simulink library "ecrobot_nxt_lib"  (Simulink 6.4)
undefined symbols (not defined in the file or in its folder): BatteryVoltage, clearNXTSignalObjects, CompassSensorS1, EnterButton, GyroSensorS1, InitAccessorBlock, InitInterfaceBlock, LightSensorS1, RevolutionSensorA, RunButton, ServoMotorA, set_fcncallname, sfunxymap2, SoundSensorS1, SoundWAV, SystemClock, TouchSensorS1, TRACK_MAP, UltrasonicSensorS1
(part 1 of 2)
settings Model: Creator=tchikama  LastModifiedBy=tchikama

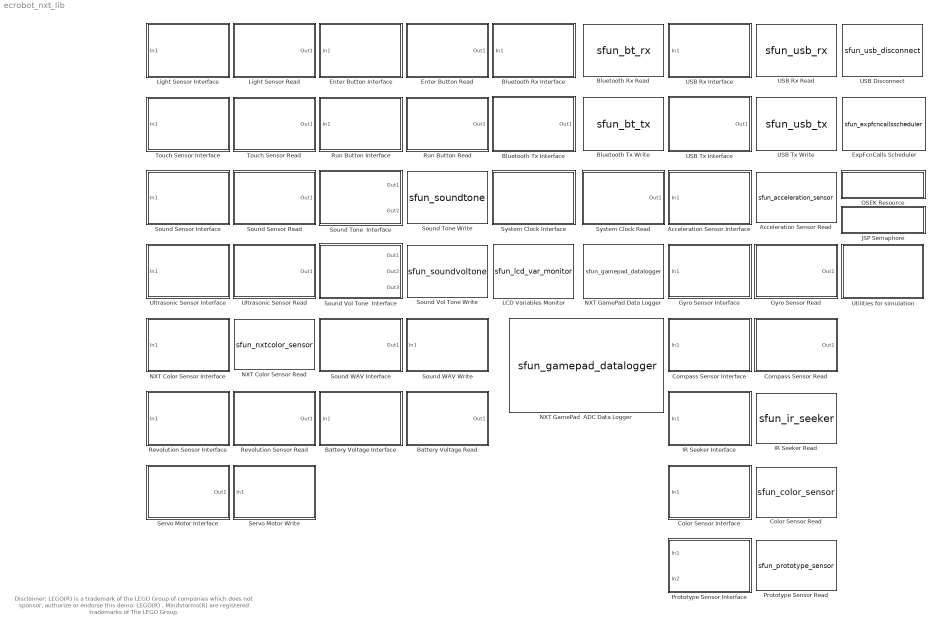
== system ecrobot_nxt_lib ==
  note: Disclaimer:
      | LEGO(R) is a trademark of the LEGO Group of companies which does not sponsor, authorize or endorse this demo.
      | LEGO(R) , Mindstorms(R) are registered trademarks of The LEGO Group.
  Acceleration Sensor Interface : Subsystem  StopFcn=clearNXTSignalObjects();  TreatAsAtomicUnit=on  mask(Acceleration Sensor Interface){ip=S1}
      mask prompts: ip "Port:"
      mask help:
      | HiTechnic Acceleration Sensor Interface for LEGO Mindstorms NXT.
      | Input is a vectorized signal:
      |  Index1: X axis acceleration
      |  Index2: Y axis acceleration
      |  Index3: Z axis acceleration
      | This block should be allocated outside of a Subsystem for RTW code generation.
      mask StyleString: popup(S1|S2|S3|S4)
      mask Display:
      | image(imread('HiTechnicSensor.jpg'))
      | port_label('input', 1, ['S' num2str(ip)])
  Acceleration Sensor Read : S-Function  FunctionName=sfun_acceleration_sensor  Parameters=-1,1,ip,bd_mode  mask(Acceleration Sensor Read){ip=S1}
      mask prompts: ip "Port:"
      mask help:
      | Read HiTechnic Acceleration Sensor data.
      | Output is a vectorized signal:
      |  Index1: X axis acceleration
      |  Index2: Y axis acceleration
      |  Index3: Z axis acceleration
      mask init:
      | bd_mode = InitDeviceSFunBlock(bdroot);
      mask StyleString: popup(S1|S2|S3|S4)
      mask Display:
      | image(imread('HiTechnicSensor.jpg'))
      | port_label('output', 1, ['S' num2str(ip)])
  Battery Voltage Interface : Subsystem  InitFcn=InitInterfaceBlock(bdroot, gcb, 'BatteryVoltage', 'Write', '');  StopFcn=clearNXTSignalObjects();  TreatAsAtomicUnit=on  mask(Battery Voltage Interface){}
      mask help:
      | Battery Voltage Interface for LEGO Mindstorms NXT.
      | This block should be allocated outside of a Subsystem for RTW code generation.
      mask init:
      | [data, map]=imread('BATTERY_VOLTAGE.gif');
      | pic=ind2rgb(data,map);
      mask Display: image(pic)
  Battery Voltage Read : Subsystem  InitFcn=InitAccessorBlock(bdroot, gcb, 'BatteryVoltage', 'Read', '');  mask(Battery Voltage Read){}
      mask help: Read LEGO Mindstorms NXT Battery Voltage data.
      mask init:
      | [data, map]=imread('BATTERY_VOLTAGE.gif');
      | pic=ind2rgb(data,map);
      | 
      | L = get_param([gcb '/Data Store Read'], 'LineHandles');
      | name = get_param(L.Outport, 'Name');
      | set_param(L.Outport, 'Name', 'BatteryVoltage_');
      mask Display: image(pic)
  Bluetooth Rx Interface : Subsystem  AncestorBlock=ecrobot_nxt_lib/Bluetooth Rx Interface  TreatAsAtomicUnit=on
      mask Type: Bluetooth Rx Interface
      mask Description:
      | Bluetooth Receive Data Packet Interface for LEGO Mindstorms NXT.
      | Size of Receive Data Packet is 32 and data type is uint8.
      | This block should be allocated outside of a Subsystem for RTW code generation and
      | should be used only single instance in a model.
      mask Display:
      | image(imread('BLUETOOTH.jpg'))
      | port_label('input', 1, 'BTRx')
  Bluetooth Rx Read : S-Function  FunctionName=sfun_bt_rx  Parameters=-1,1,bd_mode  mask(Bluetooth Rx Read){}
      mask help:
      | Read LEGO Mindstorms Bluetooth data packet. Size of data packet is 32bytes.
      | This block should be used only single instance in a model.
      mask init:
      | bd_mode = InitDeviceSFunBlock(bdroot);
      mask Display:
      | image(imread('BLUETOOTH.jpg'))
      | port_label('output', 1, 'BTRx')
  Bluetooth Tx Interface : Subsystem  AncestorBlock=ecrobot_nxt_lib/Bluetooth Tx Interface  TreatAsAtomicUnit=on
      mask Type: Bluetooth Rx Interface
      mask Description:
      | Bluetooth Send Data Packet Interface for LEGO Mindstorms NXT.
      | Size of Send Data Packet is 32 and data type is uint8.
      | This block should be allocated outside of a Subsystem for RTW code generation and
      | should be used only single instance in a model.
      mask Display:
      | image(imread('BLUETOOTH.jpg'))
      | port_label('output', 1, 'BTTx')
  Bluetooth Tx Write : S-Function  FunctionName=sfun_bt_tx  Parameters=-1,1,bd_mode  mask(Bluetooth Tx Write){}
      mask help:
      | Write LEGO Mindstorms Bluetooth data packet. Size of data packet is 32bytes.
      | This block should be used only single instance in a model.
      mask init:
      | bd_mode = InitDeviceSFunBlock(bdroot);
      mask Display:
      | image(imread('BLUETOOTH.jpg'))
      | port_label('input', 1, 'BTTx')
  Color Sensor Interface : Subsystem  AncestorBlock=ecrobot_nxt_lib/Infrared Sensor Interface  StopFcn=clearNXTSignalObjects();  TreatAsAtomicUnit=on  mask(Color Sensor Interface){ip=S1}
      mask prompts: ip "Port:"
      mask help:
      | HiTechnic Color Sensor Interface for LEGO Mindstorms NXT.
      | Input is a vectorized signal:
      |  Index1: Red color raw data
      |  Index2: Green color raw data
      |  Index3: Blue color raw data
      | This block should be allocated outside of a Subsystem for RTW code generation.
      mask StyleString: popup(S1|S2|S3|S4)
      mask Display:
      | image(imread('ColorSensor.jpeg'))
      | port_label('input', 1, ['S' num2str(ip)])
  Color Sensor Read : S-Function  AncestorBlock=ecrobot_nxt_lib/Infrared Sensor Read  FunctionName=sfun_color_sensor  Parameters=-1,1,ip,bd_mode  mask(Color Sensor Read){ip=S1}
      mask prompts: ip "Port:"
      mask help:
      | Read HiTechnic Color Sensor data.
      | Output is a vectorized signal:
      |  Index1: Red color raw data
      |  Index2: Green color raw data
      |  Index3: Blue color raw data
      mask init:
      | bd_mode = InitDeviceSFunBlock(bdroot);
      mask StyleString: popup(S1|S2|S3|S4)
      mask Display:
      | image(imread('ColorSensor.jpeg'))
      | port_label('output', 1, ['S' num2str(ip)])
  Compass Sensor Interface : Subsystem  InitFcn=InitInterfaceBlock(bdroot, gcb, 'CompassSensor', 'Write', get_param(gcb, 'ip'));  StopFcn=clearNXTSignalObjects();  TreatAsAtomicUnit=on  mask(Compass Sensor Interface){ip=S1}
      mask prompts: ip "Port:"
      mask help:
      | HiTechnic Compass Sensor Interface for LEGO Mindstorms NXT.
      | This block should be allocated outside of a Subsystem for RTW code generation.
      mask StyleString: popup(S1|S2|S3|S4)
      mask Display:
      | image(imread('HiTechnicSensor.jpg'))
      | port_label('input', 1, ip)
  Compass Sensor Read : Subsystem  InitFcn=InitAccessorBlock(bdroot, gcb, 'CompassSensor', 'Read', get_param(gcb, 'ip'));  mask(Compass Sensor Read){ip=S1}
      mask prompts: ip "Port:"
      mask help:
      | Read HiTechnic Compass Sensor data.
      | This block should be used only single instance in a model.
      mask init:
      | L = get_param([gcb '/Data Store Read'], 'LineHandles');
      | name = get_param(L.Outport, 'Name');
      | set_param(L.Outport, 'Name', ['CompassSensor_' ip]);
      mask StyleString: popup(S1|S2|S3|S4)
      mask Display:
      | image(imread('HiTechnicSensor.jpg'))
      | port_label('output', 1, ip)
  Enter Button Interface : Subsystem  InitFcn=InitInterfaceBlock(bdroot, gcb, 'EnterButton', 'Write', '');  StopFcn=clearNXTSignalObjects();  TreatAsAtomicUnit=on
      mask Type: Enter Button Interface
      mask Description:
      | Enter Button Interface for LEGO Mindstorms NXT.
      | This block should be allocated outside of a Subsystem for RTW code generation.
      mask Display: image(imread('ENTER_BUTTON.jpg'))
  Enter Button Read : Subsystem  InitFcn=InitAccessorBlock(bdroot, gcb, 'EnterButton', 'Read', '');  mask(Enter Button Read){}
      mask help: Read LEGO Mindstorms NXT Enter Button status.
      mask init:
      | L = get_param([gcb '/Data Store Read'], 'LineHandles');
      | name = get_param(L.Outport, 'Name');
      | set_param(L.Outport, 'Name', 'EnterButton_');
      mask Display: image(imread('ENTER_BUTTON.jpg'))
  ExpFcnCalls Scheduler : S-Function  AncestorBlock=lib/ExpFcnCalls Scheduler  InitFcn=set_fcncallname(gcb);  FunctionName=sfun_expfcncallsscheduler  Parameters=NUMBER_OF_FCNS, NUMBER_OF_TRIGS, TIMING_TABLE, ts  mask(Exported Function-Calls Scheduler){fcname=' ', fctrigger=[0], ts=0.001, platform=OSEK, stacksize=[512], resources=, semaphores=, bd_mode=Slave, bd_addr=}
      mask prompts: fcname "Function-Call name(i.e. 'Fcn', 'Fcn1', 'Fcn2'):"; fctrigger "Function-Call source(i.e. [0 -1 10]):"; ts "Sample time[sec]:"; stacksize "Task stack size(i.e. [512 512 512]):"; resources "OSEK Resource(i.e. 'resA', 'resB'):"; semaphores "JSP Semaphore(i.e. 'semA', 'semB'):"; bd_mode "Bluetooth device mode:"; bd_addr "Bluetooth device address(i.e. '00', '16', '53', '04', 'F1', 'B3', '00'):"
      mask help:
      | This block generates Function-Call events according to the specified initialization/periodical/event triggers in simulation.
      | This block also generate apprepreate C source to schedule RTW-EC generated C Functions in the real NXT.
      | 'Platform',  'Task stack size', and 'Resource' parameters affect only RTW-EC code generation.
      |
      | -Function-Call name: specify Function names
      | -Function-Call source: specify the Function-Call sources.
      |   0 = Initialization
      |   Number of periodical samples = Periodical execution
      |   -1 = External event triggered execution
      |  External event triggered exection is detected only at its rising edge in simulation.
      |  External event triggered execution is not supported for target deployment.
      | -Sample time[sec]: Fixed as 0.001
      | -Platform: specify run-time platform in the real NXT.
      |   OSEK: TOPPERS/ATK(OSEK) is used as the platform for RTW-EC generated C functions in multi-tasking environment
      |     JSP: TOPPERS/JSP(uITRON) is used as the platform for RTW-EC generated C functions in multi-tasking environment
      |  -Task stack size[bytes]: specify each Task (Function-Call) stack size.
      | -OSEK Resources: specify OSEK Resources
      | -JSP Semaphores: specify JSP Semaphores
      | -Bluetooth device mode: specify Bluetooth device mode as Master/Slave.
      |   'Slave' is used for NXT-PC and NXT-NXT communications. 'Master' is used for only NXT-NXT communication.
      | -Bluetooth device address: Slave device's Bluetooth device address to be paired with the Master device. Bluetooth device address consists of 7bytes hex data.
      mask init:
      | fcname = eval(['{' fcname '}']);
      | if length(fcname) ~= length(fctrigger)
      |     error('Function-Call name list and Function-Call source list are unmatch.');
      | end
      | 
      | % S-Function Parameters
      | NUMBER_OF_FCNS = length(fcname);
      | NUMBER_OF_TRIGS = length(find(fctrigger == -1));
      | TIMING_TABLE = fctrigger;
      | 
      | % diplay Function-Call configurations on the block
      | if strcmp(platform, 'OSEK')
      |     txt = '###   OSEK Tasks   ###';
      | elseif strcmp(platform, 'JSP')
      |     txt = '###   JSP Tasks   ###';
      | end
      | 
      | if strcmp('auto', simget(bdroot, 'FixedStep'))
      |     error('Exported Function-Calls Scheduler block requires FixdStep with explicit sample time');
      | else
      |     trig_i = 1;
      |     for i = 1:length(fcname)
      |         if fctrigger(i) == 0
      |             txt = [txt '\n' fcname{i} ': Init'];
      |         elseif fctrigger(i) == -1
      |             txt = [txt '\n' fcname{i} ': Trigger(' num2str(trig_i) ')'];
      |             trig_i = trig_i+1;
      |         elseif fctrigger(i) > 0
      |             txt = [txt '\n' fcname{i} ': ' num2str(fctrigger(i)*ts) ' [sec]'];
      |         end
      |     end
      | end
      | 
      | if strcmp(bd_mode, 'Master')
      |     bd_addr = eval(['{' bd_addr '}']);
      |     if length(bd_addr) ~= 7
      |         error('Bluetooth device address should consist of 7 bytes hex data.');
      |     end
      | 
      |     for i = 1:7
      |         if length(bd_addr{i}) ~= 2
      |             error('Each Bluetooth device address data should consist of 1 byte hex data.');
      |         end
      |         ch = bd_addr{i};
      |         for j = 1:2
      |             if  ~((double('0') <= double(upper(ch(j))) && double(upper(ch(j))) <= double('9')) || (double('A') <= double(upper(ch(j))) && double(upper(ch(j))) <= double('Z')))
      |                 error('Bluetooth device address data contains invalid hex data expression.');
      |             end
      |         end
      |     end
      | end
      mask StyleString: edit,edit,edit,popup(OSEK|JSP),edit,edit,edit,popup(Master|Slave),edit
      mask CallbackString:
      | |||if strcmp(get_param(gcb, 'platform'), 'OSEK')
      |     if strcmp(get_param(gcb, 'bd_mode'), 'Master')
      |         set_param(gcb, 'MaskEnableString', 'on,on,off,on,on,on,off,on,on')
      |     else
      |         set_param(gcb, 'MaskEnableString', 'on,on,off,on,on,on,off,on,off')
      |     end
      | elseif  strcmp(get_param(gcb, 'platform'), 'JSP')
      |     if strcmp(get_param(gcb, 'bd_mode'), 'Master')
      |         set_param(gcb, 'MaskEnableString', 'on,on,off,on,on,off,on,on,on')
      |     else
      |         set_param(gcb, 'MaskEnableString', 'on,on,off,on,on,off,on,on,off')
      |     end
      | end
      | ||||if strcmp(get_param(gcb, 'platform'), 'OSEK')
      |     if strcmp(get_param(gcb, 'bd_mode'), 'Master')
      |         set_param(gcb, 'MaskEnableString', 'on,on,off,on,on,on,off,on,on')
      |     else
      |         set_param(gcb, 'MaskEnableString', 'on,on,off,on,on,on,off,on,off')
      |     end
      | elseif  strcmp(get_param(gcb, 'platform'), 'JSP')
      |     if strcmp(get_param(gcb, 'bd_mode'), 'Master')
      |         set_param(gcb, 'MaskEnableString', 'on,on,off,on,on,off,on,on,on')
      |     else
      |         set_param(gcb, 'MaskEnableString', 'on,on,off,on,on,off,on,on,off')
      |     end
      | end|
      mask Display: disp(txt)
  Gyro Sensor Interface : Subsystem  AncestorBlock=ecrobot_nxt_lib/Light Sensor Interface  InitFcn=InitInterfaceBlock(bdroot, gcb, 'GyroSensor', 'Write', get_param(gcb, 'ip'));  StopFcn=clearNXTSignalObjects();  TreatAsAtomicUnit=on  mask(Gyro Sensor Interface){ip=S1}
      mask prompts: ip "Port:"
      mask help:
      | HiTechnic Gyro Sensor Interface for LEGO Mindstorms NXT.
      | This block should be allocated outside of a Subsystem for RTW code generation.
      mask StyleString: popup(S1|S2|S3|S4)
      mask Display:
      | image(imread('HiTechnicSensor.jpg'))
      | port_label('input', 1, ip)
  Gyro Sensor Read : Subsystem  AncestorBlock=ecrobot_nxt_lib/Light Sensor Read  InitFcn=InitAccessorBlock(bdroot, gcb, 'GyroSensor', 'Read', get_param(gcb, 'ip'));  mask(Gyro Sensor Read){ip=S1}
      mask prompts: ip "Port:"
      mask help:
      | Read HiTechnic Gyro Sensor data.
      | This block should be used only single instance in a model.
      mask init:
      | L = get_param([gcb '/Data Store Read'], 'LineHandles');
      | name = get_param(L.Outport, 'Name');
      | set_param(L.Outport, 'Name', ['GyroSensor_' ip]);
      mask StyleString: popup(S1|S2|S3|S4)
      mask Display:
      | image(imread('HiTechnicSensor.jpg'))
      | port_label('output', 1, ip)
  IR Seeker Interface : Subsystem  AncestorBlock=ecrobot_nxt_lib/Acceleration Sensor Interface  StopFcn=clearNXTSignalObjects();  TreatAsAtomicUnit=on  mask(IR Seeker Interface){ip=S1}
      mask prompts: ip "Port:"
      mask help:
      | HiTechnic IR Seeker Interface for LEGO Mindstorms NXT.
      | Input is a vectorized signal:
      |  Index1: Direction
      |  Index2: Intensity1
      |  Index3: Intensity2
      |  Index4: Intensity3
      |  Index5: Intensity4
      |  Index6: Intensity5
      | This block should be allocated outside of a Subsystem for RTW code generation.
      mask StyleString: popup(S1|S2|S3|S4)
      mask Display:
      | image(imread('HiTechnicSensor.jpg'))
      | port_label('input', 1, ['S' num2str(ip)])
  IR Seeker Read : S-Function  AncestorBlock=ecrobot_nxt_lib/Acceleration Sensor Read  FunctionName=sfun_ir_seeker  Parameters=-1,1,ip,bd_mode  mask(IR Seeker Read){ip=S1}
      mask prompts: ip "Port:"
      mask help:
      | Read HiTechnic IR Seeker data.
      | Output is a vectorized signal:
      |  Index1: Direction
      |  Index2: Intensity1
      |  Index3: Intensity2
      |  Index4: Intensity3
      |  Index5: Intensity4
      |  Index6: Intensity5
      mask init:
      | bd_mode = InitDeviceSFunBlock(bdroot);
      mask StyleString: popup(S1|S2|S3|S4)
      mask Display:
      | image(imread('HiTechnicSensor.jpg'))
      | port_label('output', 1, ['S' num2str(ip)])
  JSP Semaphore : Subsystem  AncestorBlock=ecrobot_nxt_lib/OSEK Resource  mask(JSP Semaphore block){semaphore=}
      mask help: One of JSP Semaphore which are specified in the Exported Function-Calls Scheduler block could be configured. Note that this block does not affect simulation, but code generation.
      mask init:
      | semaphore = get_param(gcb, 'semaphore');
      | 
      | % check the specified semaphore is defined in the Exported Function-Calls Scheduler block
      | blk = find_system(bdroot, 'regexp', 'on', ...
      |     'BlockType', 'S-Function', ...
      |     'MaskType', 'Exported Function-Calls Scheduler');
      | if ~isempty(blk)
      |     semaphores = get_param(blk, 'semaphores');
      |     semaphores = eval([ '{' semaphores{1} '}']);
      |     if ~ismember(semaphore, semaphores)
      |         error(['JSP Semaphore: ' semaphore ' is not defined in the Exported Function-Calls Scheduler block']);
      |     end
      | end
      | 
      | % write wai_sem/sig_sem API into RTW Custom Outputs and Update Code blocks
      | RTWdataOutputs = get_param([gcb '/System Outputs'], 'RTWdata');
      | RTWdataUpdate = get_param([gcb '/System Update'], 'RTWdata');
      | LINE_FEED = sprintf('\n');
      | if ~strcmp(semaphore, '<empty>')
      |     % write wai_sem into System Outputs Execution code
      |     RTWdataOutputs.Middle = [LINE_FEED '#ifdef JSP' LINE_FEED 'wai_sem( ' semaphore ' );' LINE_FEED '#endif' LINE_FEED];
      |     % write sig_sem into System Update Exit code
      |     RTWdataUpdate.Bottom =  [LINE_FEED '#ifdef JSP' LINE_FEED 'sig_sem( ' semaphore ' );' LINE_FEED '#endif' LINE_FEED];
      | else
      |     RTWdataOutputs.Middle = [LINE_FEED '#ifdef JSP' LINE_FEED LINE_FEED '#endif' LINE_FEED];
      |     RTWdataUpdate.Bottom =  [LINE_FEED '#ifdef JSP' LINE_FEED LINE_FEED '#endif' LINE_FEED];
      | end
      | set_param([gcb '/System Outputs'], 'RTWdata', RTWdataOutputs);
      | set_param([gcb '/System Update'], 'RTWdata', RTWdataUpdate);
      mask Display: disp(['Semaphore:\n' semaphore])
  LCD Variables Monitor : S-Function  FunctionName=sfun_lcd_var_monitor
      mask Type: LCD Variables Monitor
      mask Description:
      | Display sixteen input signed integer (int32) variables on the NXT LCD.
      | Inputs signals are displayed as the following format in the LCD.
      | 
      | Input01  Input02
      | Input03  Input04
      | Input05  Input06
      | Input07  Input08
      | Input09  Input10
      | Input11  Input12
      | Input13  Input14
      | Input15  Input16
      | 
      | NOTE: The fastest LCD refresh rate is appx. 24[msec]. So this block is recommended to be placed in a Function-Call Task Subsystem which is executed longer than 24[msec] period (e.g. 50[msec])
      | NOTE: This block overrides existing LCD display feature of Embedded Coder Robot NXT.
      | NOTE: This block should be used only single instance in a model.
      mask Display: image(imread('nxtlcd.jpg'))
  Light Sensor Interface : Subsystem  InitFcn=InitInterfaceBlock(bdroot, gcb, 'LightSensor', 'Write', get_param(gcb, 'ip'));  StopFcn=clearNXTSignalObjects();  TreatAsAtomicUnit=on  mask(Light Sensor Interface){ip=S1}
      mask prompts: ip "Port:"
      mask help:
      | Light Sensor Interface for LEGO Mindstorms NXT.
      | This block should be allocated outside of a Subsystem for RTW code generation.
      mask init:
      | [data, map]=imread('LIGHT_SENSOR.gif');
      | pic=ind2rgb(data,map);
      mask StyleString: popup(S1|S2|S3|S4)
      mask Display:
      | image(pic)
      | port_label('input', 1, ip)
  Light Sensor Read : Subsystem  InitFcn=InitAccessorBlock(bdroot, gcb, 'LightSensor', 'Read', get_param(gcb, 'ip'));  mask(Light Sensor Read){ip=S1}
      mask prompts: ip "Port:"
      mask help: Read LEGO Mindstorms NXT Light Sensor data.
      mask init:
      | [data, map]=imread('LIGHT_SENSOR.gif');
      | pic=ind2rgb(data,map);
      | 
      | L = get_param([gcb '/Data Store Read'], 'LineHandles');
      | name = get_param(L.Outport, 'Name');
      | set_param(L.Outport, 'Name', ['LightSensor_' ip]);
      mask StyleString: popup(S1|S2|S3|S4)
      mask Display:
      | image(pic)
      | port_label('output', 1, ip)
  NXT Color Sensor Interface : Subsystem  StopFcn=clearNXTSignalObjects();  TreatAsAtomicUnit=on  mask(NXTColor Sensor Interface){ip=S1, sensor_mode=COLORSENSOR_RGB}
      mask prompts: ip "Port:"; sensor_mode "Sensor mode:"
      mask help:
      | NXT Color Sensor Interface for LEGO Mindstorms NXT.
      | Input is varied depending on the Sensor mode.
      | LIGHTSENSOR_NONE: Light sensor with no LED light
      | LIGHTSENSOR_RED: Light sensor with red LED light
      | LIGHTSENSOR_GREEN: Light sensor with green LED light
      | LIGHTSENSOR_BLUE: Light sensor with blue LED light
      | LIGHTSENSOR_FULL: Light sensor with full (red, green and blue) LED lights
      | COLORSENSOR_ID: Color sensor returns pre-defined color ID data
      | (0=black, 1= blue, 2=green, 3=yellow, 4=orange, 5=red, 6=white, 99=unknown color)
      | Note that the color ID might be unmatch depending on measurement conditions.
      | COLORSENSOR_RGB: Color sensor returns RGB data
      |
      | This block should be allocated outside of a Subsystem for RTW code generation.
      mask init:
      | switch(sensor_mode)
      |     case 1
      |         sensor_mode_str = 'LIGHTSENSOR_NONE';
      |     case 2
      |         sensor_mode_str = 'LIGHTSENSOR_RED';
      |     case 3
      |         sensor_mode_str = 'LIGHTSENSOR_GREEN';
      |     case 4
      |         sensor_mode_str = 'LIGHTSENSOR_BLUE';
      |     case 5
      |         sensor_mode_str = 'LIGHTSENSOR_FULL';
      |     case 6
      |         sensor_mode_str = 'COLORSENSOR_ID';
      |     case 7
      |         sensor_mode_str = 'COLORSENSOR_RGB';
      |     otherwise
      |         sensor_mode_str = '';
      | end
      mask StyleString: popup(S1|S2|S3|S4),popup(LIGHTSENSOR_NONE|LIGHTSENSOR_RED|LIGHTSENSOR_GREEN|LIGHTSENSOR_BLUE|LIGHTSENSOR_FULL|COLORSENSOR_ID|COLORSENSOR_RGB)
      mask Display:
      | image(imread('cs9694.jpg'))
      | port_label('input', 1, ['S' num2str(ip)])
      | text(5,5,sensor_mode_str)
  NXT Color Sensor Read : S-Function  FunctionName=sfun_nxtcolor_sensor  Parameters=-1,1,ip,bd_mode,sensor_mode  mask(NXTColor Sensor Read){ip=S1, sensor_mode=COLORSENSOR_RGB}
      mask prompts: ip "Port:"; sensor_mode "Sensor mode:"
      mask help:
      | NXT Color Sensor Interface for LEGO Mindstorms NXT.
      |  Output is varied depending on the Sensor mode.
      | LIGHTSENSOR_NONE: Light sensor with no LED light
      | LIGHTSENSOR_RED: Light sensor with red LED light
      | LIGHTSENSOR_GREEN: Light sensor with green LED light
      | LIGHTSENSOR_BLUE: Light sensor with blue LED light
      | LIGHTSENSOR_FULL: Light sensor with full (red, green and blue) LED lights
      | COLORSENSOR_ID: Color sensor returns pre-defined color ID data
      | (0=black, 1= blue, 2=green, 3=yellow, 4=orange, 5=red, 6=white, 99=unknown color)
      | Note that the color ID might be unmatch depending on measurement conditions.
      | COLORSENSOR_RGB: Color sensor returns RGB data
      |
      | This block should be allocated outside of a Subsystem for RTW code generation.
      mask init:
      | bd_mode = InitDeviceSFunBlock(bdroot);
      | switch(sensor_mode)
      |     case 1
      |         sensor_mode_str = 'LIGHTSENSOR_NONE';
      |     case 2
      |         sensor_mode_str = 'LIGHTSENSOR_RED';
      |     case 3
      |         sensor_mode_str = 'LIGHTSENSOR_GREEN';
      |     case 4
      |         sensor_mode_str = 'LIGHTSENSOR_BLUE';
      |     case 5
      |         sensor_mode_str = 'LIGHTSENSOR_FULL';
      |     case 6
      |         sensor_mode_str = 'COLORSENSOR_ID';
      |     case 7
      |         sensor_mode_str = 'COLORSENSOR_RGB';
      |     otherwise
      |         sensor_mode_str = '';
      | end
      mask StyleString: popup(S1|S2|S3|S4),popup(LIGHTSENSOR_NONE|LIGHTSENSOR_RED|LIGHTSENSOR_GREEN|LIGHTSENSOR_BLUE|LIGHTSENSOR_FULL|COLORSENSOR_ID|COLORSENSOR_RGB)
      mask Display:
      | image(imread('cs9694.jpg'))
      | port_label('output', 1, ['S' num2str(ip)])
      | text(5,5,sensor_mode_str)
  NXT GamePad Data Logger : S-Function  FunctionName=sfun_gamepad_datalogger  Parameters=1
      mask Type: NXT GamePad Data Logger
      mask Description:
      | Send NXT internal status to NXT GamePad Data Logger.
      | NXT GamePad Data Logger has a total 32 bytes data packet.
      | 
      | NORMAL MODE:
      | data packet 0-3bytes: system tick in msec, data type U32
      | data packet 4bytes: Data1, data type S8
      | data packet 5bytes: Data2, data type S8
      | data packet 6-7bytes: battery voltage in mV, data type U16
      | data packet 8-11bytes: Servo Motor revolution at Port A, data type S32
      | data packet 12-15bytes: Servo Motor revolution at Port B, data type S32
      | data packet 16-19bytes: Servo Motor revolution at Port C, data type S32
      | data packet 20-21bytes: Analog Sensor value at Port S1, data type S16
      | data packet 22-23bytes: Analog Sensor value at Port S2, data type S16
      | data packet 24-25bytes: Analog Sensor value at Port S3, data type S16
      | data packet 26-27bytes: Analog Sensor value at Port S4, data type S16
      | data packet 28-31bytes: I2C Sensor value, data type S32
      | 
      | Data1 and Data2 can be used for logging user selected data.
      | The logged data by NXT GamePad is saved as a CSV file.
      | 
      | NOTE: This block should not be used with Bluetooth Tx Interface/Write blocks in a model and
      | should be used only single instance in a model.
      mask Display:
      | image(imread('AnalogGamePad.jpg'))
      | port_label('input', 1, 'Data1')
      | port_label('input', 2, 'Data2')
  NXT GamePad  ADC Data Logger : S-Function  FunctionName=sfun_gamepad_datalogger  Parameters=2
      mask Type: NXT GamePad ADC Data Logger
      mask Description:
      | Send NXT internal status to NXT GamePad Data Logger.
      | NXT GamePad Data Logger has a total 32 bytes data packet.
      | 
      | data packet 0-3bytes: system tick in msec, data type U32
      | data packet 4bytes: Data1, data type S8
      | data packet 5bytes: Data2, data type S8
      | data packet 6-7bytes: battery voltage in mV, data type U16
      | data packet 8-11bytes: Servo Motor revolution at Port A, data type S32
      | data packet 12-15bytes: Servo Motor revolution at Port B, data type S32
      | data packet 16-19bytes: Servo Motor revolution at Port C, data type S32
      | data packet 20-21bytes: ADC1, data type S16
      | data packet 22-23bytes: ADC2, data type S16
      | data packet 24-25bytes: ADC3, data type S16
      | data packet 26-27bytes: ADC4, data type S16
      | data packet 28-31bytes: I2C Sensor value, data type S32
      | 
      | Data1, Data2, ADC1, ADC2, ADC3, and ADC4 can be used for logging user selected data.
      | The logged data by NXT GamePad is saved as a CSV file.
      | 
      | NOTE: This block should not be used with Bluetooth Tx Interface/Write blocks in a model and
      | should be used only single instance in a model.
      mask Display:
      | image(imread('AnalogGamePad.jpg'))
      | port_label('input', 1, 'Data1')
      | port_label('input', 2, 'Data2')
      | port_label('input', 3, 'ADC1')
      | port_label('input', 4, 'ADC2')
      | port_label('input', 5, 'ADC3')
      | port_label('input', 6, 'ADC4')
  OSEK Resource : Subsystem  AncestorBlock=lib/OSEK Resource  mask(OSEK Resource block){resource=}
      mask help: One of OSEK Resources which are specified in the Exported Function-Calls Scheduler block could be configured. Note that this block does not affect simulation, but code generation.
      mask init:
      | resource = get_param(gcb, 'resource');
      | 
      | % check the specified resource is defined in the Exported Function-Calls Scheduler block
      | blk = find_system(bdroot, 'regexp', 'on', ...
      |     'BlockType', 'S-Function', ...
      |     'MaskType', 'Exported Function-Calls Scheduler');
      | if ~isempty(blk)
      |     resources = get_param(blk, 'resources');
      |     resources = eval([ '{' resources{1} '}']);
      |     if ~ismember(resource, resources)
      |         error(['OSEK Resource: ' resource ' is not defined in the Exported Function-Calls Scheduler block']);
      |     end
      | end
      | 
      | % write Get/SetResource API into RTW Custom Outputs and Update Code blocks
      | RTWdataOutputs = get_param([gcb '/System Outputs'], 'RTWdata');
      | RTWdataUpdate = get_param([gcb '/System Update'], 'RTWdata');
      | LINE_FEED = sprintf('\n');
      | %resource = get_param(gcb, 'resource');
      | if ~strcmp(resource, '<empty>')
      |     % write GetResouce into System Outputs Execution code
      |     RTWdataOutputs.Middle = [LINE_FEED '#ifdef OSEK' LINE_FEED 'GetResource( ' resource ' );' LINE_FEED '#endif' LINE_FEED];
      |     % write ReleaseResource into System Update Exit code
      |     RTWdataUpdate.Bottom =  [LINE_FEED '#ifdef OSEK' LINE_FEED 'ReleaseResource( ' resource ' );' LINE_FEED '#endif' LINE_FEED];
      | else
      |     RTWdataOutputs.Middle = [LINE_FEED '#ifdef OSEK' LINE_FEED LINE_FEED '#endif' LINE_FEED];
      |     RTWdataUpdate.Bottom =  [LINE_FEED '#ifdef OSEK' LINE_FEED LINE_FEED '#endif' LINE_FEED];
      | end
      | set_param([gcb '/System Outputs'], 'RTWdata', RTWdataOutputs);
      | set_param([gcb '/System Update'], 'RTWdata', RTWdataUpdate);
      mask Display: disp(['Resource:\n' resource])
  Prototype Sensor Interface : Subsystem  AncestorBlock=ecrobot_nxt_lib/Acceleration Sensor Interface  StopFcn=clearNXTSignalObjects();  TreatAsAtomicUnit=on  mask(Prototype Sensor Interface){ip=S1}
      mask prompts: ip "Port:"
      mask help:
      | HiTechnic Prototype Sensor Interface for LEGO Mindstorms NXT.
      | Inputs are vectorized signals.
      | A: Analog 5 inputs (0 - 1023)
      | D: Digital 6 inputs (0/1)
      | This block should be allocated outside of a Subsystem for RTW code generation.
      mask StyleString: popup(S1|S2|S3|S4)
      mask Display:
      | image(imread('t_Solderless-proto2.jpg'))
      | port_label('input', 1, ['A' '(S' num2str(ip) ')'])
      | port_label('input', 2, ['D' '(S' num2str(ip) ')'])
  Prototype Sensor Read : S-Function  FunctionName=sfun_prototype_sensor  Parameters=-1,1,ip,bd_mode,sensor_sample_time  mask(Prototype Sensor Read){ip=S1, sensor_sample_time=10}
      mask prompts: ip "Port:"; sensor_sample_time "Sensor Sample Time (4-100[msec])"
      mask help:
      | Read HiTechnic Prototype Sensor data.
      | Outputs are vectorized signals:
      | A: Analog 5 inputs (0 - 1023)
      | D: Digital 6 inputs (0/1)
      mask init:
      | if sensor_sample_time < 4 || sensor_sample_time > 100
      |     error (['Error in ' gcb ': Sensor Sample Time should be wihtin 4 - 100 [msec].']);
      | end
      | 
      | bd_mode = InitDeviceSFunBlock(bdroot);
      mask StyleString: popup(S1|S2|S3|S4),edit
      mask Display:
      | image(imread('t_Solderless-proto2.jpg'))
      | port_label('output', 1, ['A' '(S' num2str(ip) ')'])
      | port_label('output', 2, ['D' '(S' num2str(ip) ')'])
  Revolution Sensor Interface : Subsystem  InitFcn=InitInterfaceBlock(bdroot, gcb, 'RevolutionSensor', 'Write', get_param(gcb, 'ip'));  StopFcn=clearNXTSignalObjects();  TreatAsAtomicUnit=on  mask(Revolution Sensor Interface){ip=A}
      mask prompts: ip "Port:"
      mask help:
      | Motor Revolution Sensor Interface for LEGO Mindstorms NXT.
      | This block should be allocated outside of a Subsystem for RTW code generation.
      mask init:
      | [data, map]=imread('ROTATION_SENSOR.gif');
      | pic=ind2rgb(data,map);
      mask StyleString: popup(A|B|C)
      mask Display:
      | image(pic)
      | port_label('input', 1, ip)
  Revolution Sensor Read : Subsystem  InitFcn=InitAccessorBlock(bdroot, gcb,'RevolutionSensor', 'Read', get_param(gcb, 'ip'));  mask(Revolution Sensor Read){ip=A}
      mask prompts: ip "Port:"
      mask help: Read LEGO Mindstorms NXT Motor Revolution Sensor data.
      mask init:
      | [data, map]=imread('ROTATION_SENSOR.gif');
      | pic=ind2rgb(data,map);
      | 
      | L = get_param([gcb '/Data Store Read'], 'LineHandles');
      | name = get_param(L.Outport, 'Name');
      | set_param(L.Outport, 'Name', ['RevolutionSensor_' ip]);
      mask StyleString: popup(A|B|C)
      mask Display:
      | image(pic)
      | port_label('output', 1, ip)
  Run Button Interface : Subsystem  InitFcn=InitInterfaceBlock(bdroot, gcb, 'RunButton', 'Write', '');  StopFcn=clearNXTSignalObjects();  TreatAsAtomicUnit=on
      mask Type: Run Button Interface
      mask Description:
      | Run Button Interface for LEGO Mindstorms NXT.
      | This block should be allocated outside of a Subsystem for RTW code generation.
      mask Display: image(imread('RUN_BUTTON.jpg'))
  Run Button Read : Subsystem  InitFcn=InitAccessorBlock(bdroot, gcb, 'RunButton', 'Read', '');  mask(Run Button Read){}
      mask help: Read LEGO Mindstorms NXT Run Button status.
      mask init:
      | L = get_param([gcb '/Data Store Read'], 'LineHandles');
      | name = get_param(L.Outport, 'Name');
      | set_param(L.Outport, 'Name', 'RunButton_');
      mask Display: image(imread('RUN_BUTTON.jpg'))
  Servo Motor Interface : Subsystem  InitFcn=InitInterfaceBlock(bdroot, gcb, 'ServoMotor', 'Read', get_param(gcb, 'ip'), get_param(gcb, 'mode'));  StopFcn=clearNXTSignalObjects();  TreatAsAtomicUnit=on  mask(Servo Motor Interface){ip=A, mode=Brake}
      mask prompts: ip "Port:"
      mask help:
      | Servo Motor Interface for LEGO Mindstorms NXT.
      | This block should be allocated outside of a Subsystem for RTW code generation.
      mask init:
      | [data, map]=imread('SERVO_MOTOR.gif');
      | pic=ind2rgb(data,map);
      mask StyleString: popup(A|B|C),popup(Brake|Float)
      mask Display:
      | image(pic)
      | port_label('output', 1, ip)
  Servo Motor Write : Subsystem  InitFcn=InitAccessorBlock(bdroot, gcb, 'ServoMotor', 'Write', get_param(gcb, 'ip'));  mask(Servo Motor Write){ip=A}
      mask prompts: ip "Port:"
      mask help: Write LEGO Mindstorms NXT Servo Motor data.
      mask init:
      | [data, map]=imread('SERVO_MOTOR.gif');
      | pic=ind2rgb(data,map);
      mask StyleString: popup(A|B|C)
      mask Display:
      | image(pic)
      | port_label('input', 1, ip)
  Sound Sensor Interface : Subsystem  InitFcn=InitInterfaceBlock(bdroot, gcb, 'SoundSensor', 'Write', get_param(gcb, 'ip'));  StopFcn=clearNXTSignalObjects();  TreatAsAtomicUnit=on  mask(Sound Sensor Interface){ip=S1}
      mask prompts: ip "Port:"
      mask help:
      | Sound Sensor Interface for LEGO Mindstorms NXT.
      | This block should be allocated outside of a Subsystem for RTW code generation.
      mask init:
      | [data, map]=imread('SOUND_SENSOR.gif');
      | pic=ind2rgb(data,map);
      mask StyleString: popup(S1|S2|S3|S4)
      mask Display:
      | image(pic)
      | port_label('input', 1, ip)
  Sound Sensor Read : Subsystem  InitFcn=InitAccessorBlock(bdroot, gcb, 'SoundSensor', 'Read', get_param(gcb, 'ip'));  mask(Sound Sensor Read){ip=S1}
      mask prompts: ip "Port:"
      mask help: Read LEGO Mindstorms NXT Sound Sensor data.
      mask init:
      | [data, map]=imread('SOUND_SENSOR.gif');
      | pic=ind2rgb(data,map);
      | 
      | L = get_param([gcb '/Data Store Read'], 'LineHandles');
      | name = get_param(L.Outport, 'Name');
      | set_param(L.Outport, 'Name', ['SoundSensor_' ip]);
      mask StyleString: popup(S1|S2|S3|S4)
      mask Display:
      | image(pic)
      | port_label('output', 1, ip)
  Sound Tone Write : S-Function  FunctionName=sfun_soundtone  Parameters=-1,1,bd_mode  mask(Sound Tone Write){}
      mask help:
      | Write LEGO Mindstorms NXT Sound Tone data.
      |
      | Freq: Frequency of a tone sound in Hertz (Hz)
      | Dur: Duration of a tone sound, in centiseconds. Value is truncated at 256 centiseconds
      mask init:
      | bd_mode = InitDeviceSFunBlock(bdroot);
      mask Display:
      | image(imread('BEEP.jpg'))
      | port_label('input', 1, 'Freq')
      | port_label('input', 2, 'Dur')
  Sound Tone  Interface : Subsystem  TreatAsAtomicUnit=on
      mask Type: Sound Tone Interface
      mask Description:
      | Sound Tone Interface for LEGO Mindstorms NXT.
      | This block should be allocated outside of a Subsystem for RTW code generation and
      | should be used only single instance in a model.
      | 
      | Freq: Frequency of a tone sound in Hertz (Hz)
      | Dur: Duration of a tone sound in centiseconds. Value is truncated at 256 centiseconds
      mask Display:
      | image(imread('BEEP.jpg'))
      | port_label('output', 1, 'Freq')
      | port_label('output', 2, 'Dur')
  Sound Vol Tone Write : S-Function  AncestorBlock=ecrobot_nxt_lib/Sound Tone Write  FunctionName=sfun_soundvoltone  Parameters=-1,1,bd_mode  mask(Sound Vol Tone Write){}
      mask help:
      | Write LEGO Mindstorms NXT Sound Tone data with volume.
      |
      | Freq: Frequency of a tone sound in Hertz (Hz)
      | Dur: Duration of a tone sound, in centiseconds. Value is truncated at 256 centiseconds
      | Vol: Volume of a tone sound. 0[%] to 100[%]. 0[%] means mute.
      mask init:
      | bd_mode = InitDeviceSFunBlock(bdroot);
      mask Display:
      | image(imread('BEEP.jpg'))
      | port_label('input', 1, 'Freq')
      | port_label('input', 2, 'Dur')
      | port_label('input', 3, 'Vol')
  Sound Vol Tone  Interface : Subsystem  AncestorBlock="ecrobot_nxt_lib/Sound Tone  Interface"  TreatAsAtomicUnit=on
      mask Type: Sound Vol Tone Interface
      mask Description:
      | Sound Vol Tone Interface for LEGO Mindstorms NXT.
      | This block should be allocated outside of a Subsystem for RTW code generation and
      | should be used only single instance in a model.
      | 
      | Freq: Frequency of a tone sound in Hertz (Hz)
      | Dur: Duration of a tone sound, in centiseconds. Value is truncated at 256 centiseconds
      | Vol: Volume of a tone sound. 0[%] to 100[%]. 0[%] means mute.
      mask Display:
      | image(imread('BEEP.jpg'))
      | port_label('output', 1, 'Freq')
      | port_label('output', 2, 'Dur')
      | port_label('output', 3, 'Vol')
  Sound WAV Interface : Subsystem  AncestorBlock=ecrobot_nxt_lib/Servo Motor Interface  InitFcn=InitInterfaceBlock(bdroot, gcb, 'SoundWAV', 'Read', eval(get_param(gcb, 'wav')));  StopFcn=clearNXTSignalObjects();  TreatAsAtomicUnit=on  mask(Sound WAV Interface){wav=}
      mask prompts: wav "WAV file name (e.g. 'mtlb'):"
      mask help:
      | Sound WAV Interface for LEGO Mindstorms NXT.
      | This block should be allocated outside of a Subsystem for RTW code generation.
      | Support for only 2k - 22 kHz 8bit monoral WAV file.
      |
      | Vol: Volume of a WAV sound. 0[%] to 100[%]. 0[%] means mute
      mask init:
      | wavfile = [wav '.wav'];
      | if isempty(which(wavfile));
      |     error ([wav ' is invalid file name or does not exist in MATLAB path.']);
      | end
      mask Display:
      | disp(wavfile);
      | port_label('output', 1, 'Vol')
  Sound WAV Write : Subsystem  AncestorBlock=ecrobot_nxt_lib/Servo Motor Write  InitFcn=InitAccessorBlock(bdroot, gcb, 'SoundWAV', 'Write', eval(get_param(gcb, 'wav')));  mask(Sound WAV Write){wav=}
      mask prompts: wav "WAV file name (e.g. 'mtlb'):"
      mask help:
      | Write LEGO Mindstorms NXT Sound WAV volume data.
      | Support for only 2k - 22 kHz 8bit monoral WAV file.
      |
      | Vol: Volume of a WAV sound. 0[%] to 100[%]. 0[%] means mute.
      mask init:
      | wavfile = [wav '.wav'];
      | if isempty(which(wavfile));
      |     error ([wav ' is invalid file name or does not exist in MATLAB path.']);
      | end
      mask Display:
      | disp(wavfile);
      | port_label('input', 1, 'Vol')
  System Clock Interface : Subsystem  InitFcn=InitInterfaceBlock(bdroot, gcb, 'SystemClock', 'Write', '');  StopFcn=clearNXTSignalObjects();  TreatAsAtomicUnit=on  mask(System Clock Interface){}
      mask help:
      | System Clock Interface for LEGO Mindstorms NXT.
      | This block should be allocated outside of a Subsystem for RTW code generation.
      mask init:
      | [data, map]=imread('SYSTEM_CLOCK.gif');
      | pic=ind2rgb(data,map);
      mask Display: image(pic)
  System Clock Read : Subsystem  InitFcn=InitAccessorBlock(bdroot, gcb, 'SystemClock', 'Read', '');  mask(System Clock Read){}
      mask help: Read LEGO Mindstorms NXT System Clock data.
      mask init:
      | [data, map]=imread('SYSTEM_CLOCK.gif');
      | pic=ind2rgb(data,map);
      | 
      | L = get_param([gcb '/Data Store Read'], 'LineHandles');
      | name = get_param(L.Outport, 'Name');
      | set_param(L.Outport, 'Name', 'SystemClock_');
      mask Display: image(pic)
  Touch Sensor Interface : Subsystem  InitFcn=InitInterfaceBlock(bdroot, gcb, 'TouchSensor', 'Write', get_param(gcb, 'ip'));  StopFcn=clearNXTSignalObjects();  TreatAsAtomicUnit=on  mask(Touch Sensor Interface){ip=S1}
      mask prompts: ip "Port:"
      mask help:
      | Touch Sensor Interface for LEGO Mindstorms NXT.
      | This block should be allocated outside of a Subsystem for RTW code generation.
      mask init:
      | [data, map]=imread('TOUCH_SENSOR.gif');
      | pic=ind2rgb(data,map);
      mask StyleString: popup(S1|S2|S3|S4)
      mask Display:
      | image(pic)
      | port_label('input', 1, ip)
  Touch Sensor Read : Subsystem  InitFcn=InitAccessorBlock(bdroot, gcb, 'TouchSensor', 'Read', get_param(gcb, 'ip'));  mask(Touch Sensor Read){ip=S1}
      mask prompts: ip "Port:"
      mask help: Read LEGO Mindstorms NXT Touch Sensor data.
      mask init:
      | [data, map]=imread('TOUCH_SENSOR.gif');
      | pic=ind2rgb(data,map);
      | 
      | L = get_param([gcb '/Data Store Read'], 'LineHandles');
      | name = get_param(L.Outport, 'Name');
      | set_param(L.Outport, 'Name', ['TouchSensor_' ip]);
      mask StyleString: popup(S1|S2|S3|S4)
      mask Display:
      | image(pic)
      | port_label('output', 1, ip)
  USB Disconnect : S-Function  FunctionName=sfun_usb_disconnect
      mask Type: USB Disconnect
      mask Description: Disconnect a USB connection with the host device.
      mask Display:
      | image(imread('usb1394_02_r.jpg'))
      | port_label('input', 1, 'Disconnect')
  USB Rx Interface : Subsystem  AncestorBlock=ecrobot_nxt_lib/Bluetooth Rx Interface  TreatAsAtomicUnit=on
      mask Type: USB Rx Interface
      mask Description:
      | USB Receive Data Packet Interface for LEGO Mindstorms NXT.
      | Size of Receive Data Packet is 64 and data type is uint8.
      | This block should be allocated outside of a Subsystem for RTW code generation and
      | should be used only single instance in a model.
      mask Display:
      | image(imread('usb1394_02_l.jpg'))
      | port_label('input', 1, 'USBRx')
  USB Rx Read : S-Function  AncestorBlock=ecrobot_nxt_lib/Bluetooth Rx Read  FunctionName=sfun_usb_rx  Parameters=-1,1,bd_mode  mask(USB Rx Read){}
      mask help:
      | Read LEGO Mindstorms USB data packet. Size of data packet is 64bytes.
      | This block should be used only single instance in a model.
      mask init:
      | bd_mode = InitDeviceSFunBlock(bdroot);
      mask Display:
      | image(imread('usb1394_02_l.jpg'))
      | port_label('output', 1, 'USBRx')
  USB Tx Interface : Subsystem  AncestorBlock=ecrobot_nxt_lib/Bluetooth Tx Interface  TreatAsAtomicUnit=on
      mask Type: USB Rx Interface
      mask Description:
      | USB Send Data Packet Interface for LEGO Mindstorms NXT.
      | Size of Send Data Packet is 64 and data type is uint8.
      | This block should be allocated outside of a Subsystem for RTW code generation and
      | should be used only single instance in a model.
      mask Display:
      | image(imread('usb1394_02_r.jpg'))
      | port_label('output', 1, 'USBTx')
  USB Tx Write : S-Function  AncestorBlock=ecrobot_nxt_lib/Bluetooth Tx Write  FunctionName=sfun_usb_tx  Parameters=-1,1,bd_mode  mask(USB Tx Write){}
      mask help:
      | Write LEGO Mindstorms USB data packet. Size of data packet is 64bytes.
      | This block should be used only single instance in a model.
      mask init:
      | bd_mode = InitDeviceSFunBlock(bdroot);
      mask Display:
      | image(imread('usb1394_02_r.jpg'))
      | port_label('input', 1, 'USBTx')
  Ultrasonic Sensor Interface : Subsystem  InitFcn=InitInterfaceBlock(bdroot, gcb, 'UltrasonicSensor', 'Write', get_param(gcb, 'ip'));  StopFcn=clearNXTSignalObjects();  TreatAsAtomicUnit=on  mask(Ultrasonic Sensor Interface){ip=S1}
      mask prompts: ip "Port:"
      mask help:
      | Ultrasonic Sensor Interface for LEGO Mindstorms NXT.
      | This block should be allocated outside of a Subsystem for RTW code generation.
      mask init:
      | [data, map]=imread('SONIC_SENSOR.gif');
      | pic=ind2rgb(data,map);
      mask StyleString: popup(S1|S2|S3|S4)
      mask Display:
      | image(pic)
      | port_label('input', 1, ip)
  Ultrasonic Sensor Read : Subsystem  InitFcn=InitAccessorBlock(bdroot, gcb, 'UltrasonicSensor', 'Read', get_param(gcb, 'ip'));  mask(Ultrasonic Sensor Read){ip=S1}
      mask prompts: ip "Port:"
      mask help: Read LEGO Mindstorms NXT Ultrasonic Sensor data.
      mask init:
      | [data, map]=imread('SONIC_SENSOR.gif');
      | pic=ind2rgb(data,map);
      | 
      | L = get_param([gcb '/Data Store Read'], 'LineHandles');
      | name = get_param(L.Outport, 'Name');
      | set_param(L.Outport, 'Name', ['UltrasonicSensor_' ip]);
      mask StyleString: popup(S1|S2|S3|S4)
      mask Display:
      | image(pic)
      | port_label('output', 1, ip)
  Utilities for simulation : Subsystem
      mask Display: disp('Utilities')

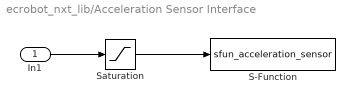
== system ecrobot_nxt_lib/Acceleration Sensor Interface ==
  In1 : Inport
  S-Function : S-Function  FunctionName=sfun_acceleration_sensor  Parameters=0.001,0,ip,bd_mode
      mask init:
      | bd_mode = InitDeviceSFunBlock(bdroot);
  Saturation : Saturate  UpperLimit=511  LowerLimit=-512
  wires:
  In1/1 -> Saturation/1
  Saturation/1 -> S-Function/1

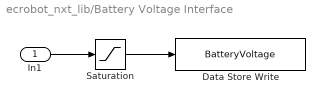
== system ecrobot_nxt_lib/Battery Voltage Interface ==
  In1 : Inport
  Data Store Write : DataStoreWrite  DataStoreName=BatteryVoltage  SampleTime=0.001
  Saturation : Saturate  UpperLimit=BatteryVoltage.Max  LowerLimit=BatteryVoltage.Min  SampleTime=0.001
  wires:
  Saturation/1 -> Data Store Write/1
  In1/1 -> Saturation/1

== system ecrobot_nxt_lib/Battery Voltage Read ==
  Data Store Read : DataStoreRead  DataStoreName=BatteryVoltage  SampleTime=-1
  Out1 : Outport
  wires:
  Data Store Read/1 -> Out1/1  "BatteryVoltage_"

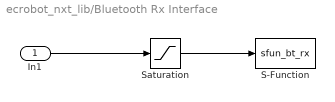
== system ecrobot_nxt_lib/Bluetooth Rx Interface ==
  In1 : Inport
  S-Function : S-Function  FunctionName=sfun_bt_rx  Parameters=0.001,0,bd_mode
      mask init:
      | bd_mode = InitDeviceSFunBlock(bdroot);
  Saturation : Saturate  UpperLimit=255  LowerLimit=0
  wires:
  Saturation/1 -> S-Function/1
  In1/1 -> Saturation/1

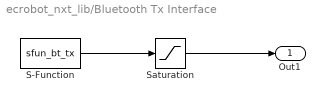
== system ecrobot_nxt_lib/Bluetooth Tx Interface ==
  S-Function : S-Function  FunctionName=sfun_bt_tx  Parameters=0.001,0,bd_mode
      mask init:
      | bd_mode = InitDeviceSFunBlock(bdroot);
  Saturation : Saturate  UpperLimit=255  LowerLimit=0
  Out1 : Outport
  wires:
  Saturation/1 -> Out1/1
  S-Function/1 -> Saturation/1

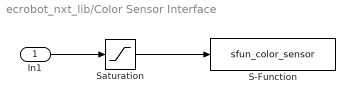
== system ecrobot_nxt_lib/Color Sensor Interface ==
  In1 : Inport
  S-Function : S-Function  FunctionName=sfun_color_sensor  Parameters=0.001,0,ip,bd_mode
      mask init:
      | bd_mode = InitDeviceSFunBlock(bdroot);
  Saturation : Saturate  UpperLimit=1023  LowerLimit=0
  wires:
  In1/1 -> Saturation/1
  Saturation/1 -> S-Function/1

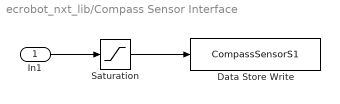
== system ecrobot_nxt_lib/Compass Sensor Interface ==
  In1 : Inport
  Data Store Write : DataStoreWrite  DataStoreName=CompassSensorS1  SampleTime=0.001
  Saturation : Saturate  UpperLimit=CompassSensorS1.Max  LowerLimit=CompassSensorS1.Min  SampleTime=0.001
  wires:
  In1/1 -> Saturation/1
  Saturation/1 -> Data Store Write/1

== system ecrobot_nxt_lib/Compass Sensor Read ==
  Data Store Read : DataStoreRead  DataStoreName=CompassSensorS1  SampleTime=-1
  Out1 : Outport
  wires:
  Data Store Read/1 -> Out1/1  "CompassSensor_S1"

== system ecrobot_nxt_lib/Enter Button Interface ==
  In1 : Inport
  Data Store Write : DataStoreWrite  DataStoreName=EnterButton  SampleTime=0.001
  Saturation : Saturate  UpperLimit=EnterButton.Max  LowerLimit=EnterButton.Min  SampleTime=0.001
  wires:
  In1/1 -> Saturation/1
  Saturation/1 -> Data Store Write/1

== system ecrobot_nxt_lib/Enter Button Read ==
  Data Store Read : DataStoreRead  DataStoreName=BatteryVoltage  SampleTime=-1
  Out1 : Outport
  wires:
  Data Store Read/1 -> Out1/1  "EnterButton_"

== system ecrobot_nxt_lib/Gyro Sensor Interface ==
  In1 : Inport
  Data Store Write : DataStoreWrite  DataStoreName=GyroSensorS1  SampleTime=0.001
  Saturation : Saturate  UpperLimit=GyroSensorS1.Max  LowerLimit=GyroSensorS1.Min  SampleTime=0.001
  wires:
  Saturation/1 -> Data Store Write/1
  In1/1 -> Saturation/1

== system ecrobot_nxt_lib/Gyro Sensor Read ==
  Data Store Read : DataStoreRead  DataStoreName=LightSensorS1  SampleTime=-1
  Out1 : Outport
  wires:
  Data Store Read/1 -> Out1/1  "GyroSensor_S1"

== system ecrobot_nxt_lib/IR Seeker Interface ==
  In1 : Inport
  S-Function : S-Function  FunctionName=sfun_ir_seeker  Parameters=0.001,0,ip,bd_mode
      mask init:
      | bd_mode = InitDeviceSFunBlock(bdroot);
  Saturation : Saturate  UpperLimit=127  LowerLimit=-128
  wires:
  Saturation/1 -> S-Function/1
  In1/1 -> Saturation/1
